simulink model "Lab_5_pend_est"  (R2018a)
settings: Solver=VariableStepAuto  StartTime=0.0  StopTime=10.0  RelTol=1e-3
undefined symbols (not defined in the file): c, g, L, m, theta0
settings Model: Creator=Patrick  LastModifiedBy=Patrick

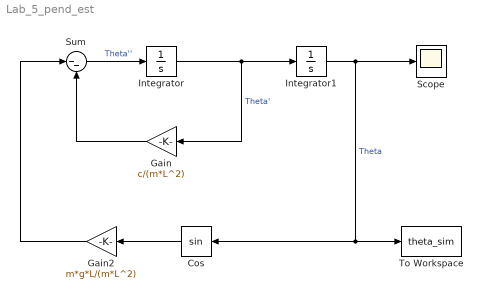
== system Lab_5_pend_est ==
  Cos : Trigonometry
  Gain : Gain  Gain=c/(m*L^2)
  Gain2 : Gain  Gain=m*g*L/(m*L^2)
  Integrator : Integrator
  Integrator1 : Integrator  InitialCondition=theta0
  Scope : Scope
  Sum : Sum  Inputs=|--
  To Workspace : ToWorkspace  VariableName=theta_sim  SaveFormat=Timeseries  SampleTime=-1
  wires:
  Gain/1 -> Sum/2
  Integrator/1 -> Gain/1, Integrator1/1  "Theta'"
  Sum/1 -> Integrator/1  "Theta''"
  Gain2/1 -> Sum/1
  Cos/1 -> Gain2/1
  Integrator1/1 -> Scope/1, To Workspace/1, Cos/1  "Theta"
